simulink model "PVGRIDup2018"  (R2018a)
settings: Solver=VariableStepAuto  StartTime=0.0  StopTime=1  FixedStep=6.17283950617284E-7  MaxStep=2.0E-5  RelTol=1e-3
libraries: powerlib x33, powerlib_meascontrol x5, fuzblock x2, powerlib_extras x2, simulink x2, eePowerMeasurement x1, re_lib x1
(part 1 of 2)
settings Model: Creator=Lenovo  LastModifiedBy=Lenovo
settings SolverCC: AlgebraicLoopSolver=LineSearch
settings DataIOCC: ReturnWorkspaceOutputs=on
settings SFSimCC: SimUseLocalCustomCode=on
settings RTWCC: RTWUseLocalCustomCode=on

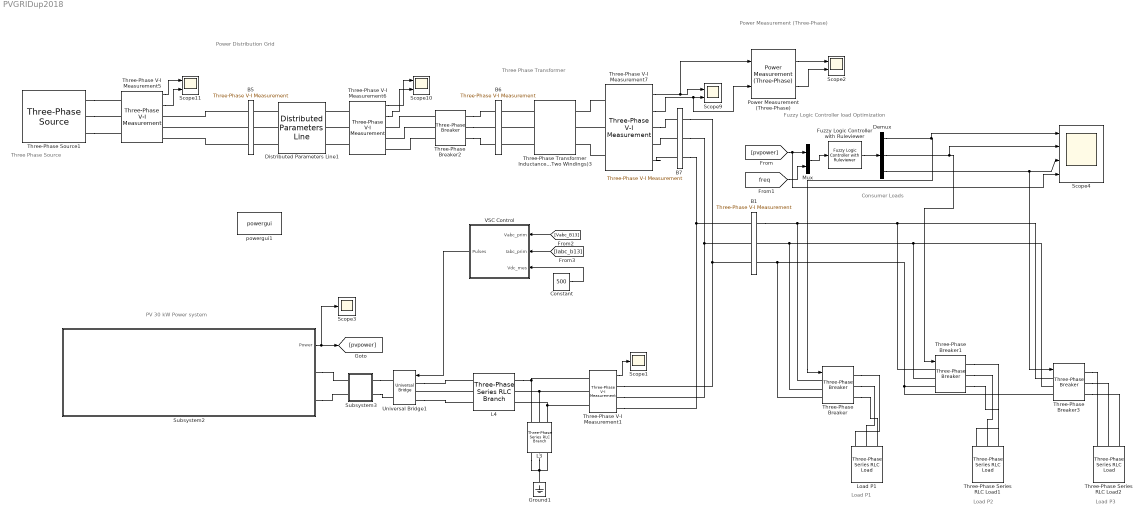
== system PVGRIDup2018 ==
  note: Fuzzy Logic Controller load Optimization
  note: Power Measurement
      | (Three-Phase)
  note: Three Phase Transformer
  note: Three Phase Source
  note: PV 30 kW Power system
  note: Load P1
  note: Power Distribution Grid
  note: Load P2
  note: Load P3
  note: Consumer Loads
  B1 : powerlib/Measurements/Three-Phase V-I Measurement  VoltageMeasurement=no  SetLabelV=off  LabelV=Vabc_B13  Vpu=off  VpuLL=off  CurrentMeasurement=no  SetLabelI=off  LabelI=Iabc_b13  Ipu=off  Pbase=100e6  Vbase=440  OutputType=Magnitude  PhasorSimulation=off  PSBequivalent=0
  B5 : powerlib/Measurements/Three-Phase V-I Measurement  VoltageMeasurement=no  SetLabelV=off  LabelV=Vabc_B12  Vpu=off  VpuLL=off  CurrentMeasurement=no  SetLabelI=off  LabelI=A1  Ipu=off  Pbase=100e6  Vbase=25e3  OutputType=Magnitude  PhasorSimulation=off  PSBequivalent=0
  B6 : powerlib/Measurements/Three-Phase V-I Measurement  VoltageMeasurement=no  SetLabelV=off  LabelV=Vabc_B12  Vpu=off  VpuLL=off  CurrentMeasurement=no  SetLabelI=off  LabelI=A1  Ipu=off  Pbase=100e6  Vbase=440  OutputType=Magnitude  PhasorSimulation=off  PSBequivalent=0
  B7 : powerlib/Measurements/Three-Phase V-I Measurement  VoltageMeasurement=phase-to-ground  SetLabelV=on  LabelV=Vabc_B13  Vpu=off  VpuLL=off  CurrentMeasurement=yes  SetLabelI=on  LabelI=Iabc_b13  Ipu=off  Pbase=100e6  Vbase=440  OutputType=Magnitude  PhasorSimulation=off  PSBequivalent=0
  Constant : Constant  Value=500
  Demux : Demux  Outputs=3
  Distributed Parameters Line1 : powerlib/Elements/Distributed Parameters Line  Phases=3  Frequency=50  Resistance=[0.01273 0.3864]  Inductance="[0.9337e-3  4.1264e-3]"  Capacitance=[12.74e-9 7.751e-9]  Length=100  x1=[-0.000566 5.83136712290493e-10 21736.6395103712 -60787.0989053576;-0.000565 5.82440364018513e-10 21755.7352677324 -60780.2671390469;-0.000564 5.81743958261973e-10 21774.8288778885 -60773.4293739643;-0.000563 5.81047495089606e-10 21793.9203389552 -60766.5856107847;-0.000562 5.8035097457015e-10 21813.0096490482 -60759.7358501836;-0.000561 5.7965439677235e-10 21832.0968062834 -60752.8800928369;-0.00056 5.78957761764954e-10 21851.1818087771 -60746.0183394214;-0.000559 5.78261069616718e-10 21870.2646546456 -60739.1505906142;-0.000558 5.77564320396403e-10 21889.3453420055 -60732.2768470932;-0.000557 5.76867514172774e-10 21908.4238689736 -60725.3971095368;-0.000556 5.76170651014605e-10 21927.500233667 -60718.511378624;-0.000555 5.75473730990671e-10 21946.5744342028 -60711.6196550343;-0.000554 5.74776754169758e-10 21965.6464686987 -60704.721939448;-0.000553 5.74079720620653e-10 21984.7163352721 -60697.8182325458;-0.000552 5.73382630412152e-10 22003.784032041 -60690.9085350092;-0.000551 5.72685483613053e-10 22022.8495571235 -60683.99284752;-0.00055 5.71988280292163e-10 22041.9129086378 -60677.0711707608;-0.000549 5.71291020518294e-10 22060.9740847026 -60670.1435054148;-0.000548 5.70593704360261e-10 22080.0330834366 -60663.2098521657;-0.000547 5.69896331886887e-10 22099.0899029586 -60656.2702116979;-0.000546 5.69198903167e-10 22118.1445413879 -60649.3245846961;-0.000545 5.68501418269433e-10 22137.1969968438 -60642.372971846;-0.000544 5.67803877263027e-10 22156.2472674461 -60635.4153738336;-0.000543 5.67106280216624e-10 22175.2953513143 -60628.4517913457;-0.000542 5.66408627199075e-10 22194.3412465687 -60621.4822250694;-0.000541 5.65710918279236e-10 22213.3849513294 -60614.5066756928;-0.00054 5.65013153525967e-10 22232.4264637169 -60607.5251439041;-0.000539 5.64315333008136e-10 22251.4657818518 -60600.5376303926;-0.000538 5.63617456794614e-10 22270.5029038552 -60593.5441358477;-0.000537 5.6291952495428e-10 22289.537827848 -60586.5446609599;-0.000536 5.62221537556016e-10 22308.5705519516 -60579.5392064197;-0.000535 5.61523494668711e-10 22327.6010742876 -60572.5277729188;-0.000534 5.60825396361258e-10 22346.6293929778 -60565.510361149;-0.000533 5.60127242702558e-10 22365.655506144 -60558.4869718031;-0.000532 5.59429033761516e-10 22384.6794119085 -60551.457605574;-0.000531 5.58730769607041e-10 22403.7011083937 -60544.4222631557;-0.00053 5.5803245030805e-10 22422.7205937223 -60537.3809452425;-0.000529 5.57334075933465e-10 22441.7378660171 -60530.3336525293;-0.000528 5.56635646552211e-10 22460.7529234011 -60523.2803857117;-0.000527 5.55937162233222e-10 22479.7657639977 -60516.2211454858;-0.000526 5.55238623045434e-10 22498.7763859304 -60509.1559325483;-0.000525 5.54540029057792e-10 22517.7847873228 -60502.0847475966;-0.000524 5.53841380339242e-10 22536.7909662991 -60495.0075913285;-0.000523 5.5314267695874e-10 22555.7949209832 -60487.9244644425;-0.000522 5.52443918985244e-10 22574.7966494996 -60480.8353676377;-0.000521 5.5174510648772e-10 22593.7961499729 -60473.7403016137;-0.00052 5.51046239535136e-10 22612.7934205279 -60466.6392670709;-0.000519 5.50347318196469e-10 22631.7884592897 -60459.53226471;-0.000518 5.496483425407e-10 22650.7812643835 -60452.4192952325;-0.000517 5.48949312636813e-10 22669.7718339348 -60445.3003593405;-0.000516 5.48250228553802e-10 22688.7601660693 -60438.1754577364;-0.000515 5.47551090360663e-10 22707.746258913 -60431.0445911236;-0.000514 5.46851898126397e-10 22726.730110592 -60423.9077602058;-0.000513 5.46152651920013e-10 22745.7117192326 -60416.7649656874;-0.000512 5.45453351810523e-10 22764.6910829615 -60409.6162082733;-0.000511 5.44753997866946e-10 22783.6681999055 -60402.4614886692;-0.00051 5.44054590158304e-10 22802.6430681915 -60395.3008075811;-0.000509 5.43355128753627e-10 22821.615685947 -60388.1341657157;-0.000508 5.42655613721949e-10 22840.5860512992 -60380.9615637805;-0.000507 5.41956045132309e-10 22859.554162376 -60373.7830024833;-0.000506 5.41256423053752e-10 22878.5200173052 -60366.5984825326 ...(+32961 chars)]  x2=[-0.000566 3.58367798971719e-09 21848.8110670649 -61151.5428268991;-0.000565 3.58079247310706e-09 21868.0213123234 -61144.6758028705;-0.000564 3.57790660308688e-09 21887.2293992947 -61137.8027441044;-0.000563 3.57502037994147e-09 21906.435326083 -61130.9236512791;-0.000562 3.5721338039557e-09 21925.6390907929 -61124.0385250735;-0.000561 3.56924687541445e-09 21944.8406915289 -61117.1473661671;-0.00056 3.56635959460267e-09 21964.040126396 -61110.2501752401;-0.000559 3.5634719618053e-09 21983.2373934992 -61103.3469529733;-0.000558 3.56058397730735e-09 22002.4324909439 -61096.4377000478;-0.000557 3.55769564139384e-09 22021.6254168355 -61089.5224171457;-0.000556 3.55480695434986e-09 22040.8161692799 -61082.6011049495;-0.000555 3.5519179164605e-09 22060.0047463829 -61075.6737641422;-0.000554 3.54902852801089e-09 22079.1911462508 -61068.7403954076;-0.000553 3.5461387892862e-09 22098.3753669898 -61061.80099943;-0.000552 3.54324870057165e-09 22117.5574067066 -61054.8555768941;-0.000551 3.54035826215248e-09 22136.737263508 -61047.9041284857;-0.00055 3.53746747431395e-09 22155.9149355011 -61040.9466548906;-0.000549 3.53457633734138e-09 22175.090420793 -61033.9831567957;-0.000548 3.53168485152011e-09 22194.2637174912 -61027.0136348881;-0.000547 3.52879301713552e-09 22213.4348237034 -61020.0380898557;-0.000546 3.52590083447302e-09 22232.6037375375 -61013.0565223871;-0.000545 3.52300830381806e-09 22251.7704571016 -61006.0689331711;-0.000544 3.52011542545612e-09 22270.934980504 -60999.0753228975;-0.000543 3.51722219967272e-09 22290.0973058532 -60992.0756922566;-0.000542 3.5143286267534e-09 22309.257431258 -60985.0700419391;-0.000541 3.51143470698375e-09 22328.4153548274 -60978.0583726366;-0.00054 3.5085404406494e-09 22347.5710746705 -60971.0406850409;-0.000539 3.50564582803598e-09 22366.7245888968 -60964.0169798448;-0.000538 3.50275086942919e-09 22385.8758956158 -60956.9872577414;-0.000537 3.49985556511475e-09 22405.0249929375 -60949.9515194246;-0.000536 3.49695991537841e-09 22424.1718789719 -60942.9097655887;-0.000535 3.49406392050597e-09 22443.3165518293 -60935.8619969288;-0.000534 3.49116758078324e-09 22462.4590096201 -60928.8082141404;-0.000533 3.48827089649608e-09 22481.599250455 -60921.7484179197;-0.000532 3.4853738679304e-09 22500.7372724451 -60914.6826089635;-0.000531 3.4824764953721e-09 22519.8730737015 -60907.6107879691;-0.00053 3.47957877910715e-09 22539.0066523355 -60900.5329556346;-0.000529 3.47668071942154e-09 22558.1380064587 -60893.4491126584;-0.000528 3.4737823166013e-09 22577.2671341829 -60886.3592597398;-0.000527 3.4708835709325e-09 22596.3940336202 -60879.2633975784;-0.000526 3.46798448270121e-09 22615.5187028829 -60872.1615268746;-0.000525 3.46508505219359e-09 22634.6411400833 -60865.0536483293;-0.000524 3.46218527969577e-09 22653.7613433342 -60857.9397626441;-0.000523 3.45928516549397e-09 22672.8793107485 -60850.819870521;-0.000522 3.45638470987441e-09 22691.9950404393 -60843.6939726627;-0.000521 3.45348391312336e-09 22711.10853052 -60836.5620697726;-0.00052 3.45058277552711e-09 22730.2197791042 -60829.4241625546;-0.000519 3.44768129737199e-09 22749.3287843055 -60822.280251713;-0.000518 3.44477947894437e-09 22768.4355442382 -60815.1303379531;-0.000517 3.44187732053065e-09 22787.5400570164 -60807.9744219805;-0.000516 3.43897482241725e-09 22806.6423207545 -60800.8125045013;-0.000515 3.43607198489065e-09 22825.7423335672 -60793.6445862226;-0.000514 3.43316880823734e-09 22844.8400935696 -60786.4706678517;-0.000513 3.43026529274385e-09 22863.9355988766 -60779.2907500966;-0.000512 3.42736143869675e-09 22883.0288476036 -60772.1048336661;-0.000511 3.42445724638263e-09 22902.1198378662 -60764.9129192692;-0.00051 3.42155271608814e-09 22921.2085677802 -60757.7150076159;-0.000509 3.41864784809993e-09 22940.2950354616 -60750.5110994165;-0.000508 3.4157426427047e-09 22959.3792390266 -60743.3011953821;-0.000507 3.4128371001892e-09 22978.4611765918 -60736.0852962241;-0.000506 3.40993122084017e-09 22997.5408462738 -60728.8634026549 ...(+32986 chars)]  x3=[-0.000566 5.56062289169838e-11 55.6303279385759 -232.444239909909;-0.000565 5.56073424095848e-11 55.7033497037751 -232.426751656576;-0.000564 5.56084504139612e-11 55.7763659712741 -232.409240463642;-0.000563 5.56095529300035e-11 55.8493767338664 -232.391706332836;-0.000562 5.5610649957603e-11 55.9223819843462 -232.374149265888;-0.000561 5.56117414966513e-11 55.9953817155082 -232.356569264532;-0.00056 5.56128275470409e-11 56.0683759201476 -232.338966330501;-0.000559 5.56139081086644e-11 56.1413645910601 -232.321340465533;-0.000558 5.56149831814152e-11 56.2143477210421 -232.303691671369;-0.000557 5.56160527651872e-11 56.2873253028904 -232.286019949749;-0.000556 5.56171168598749e-11 56.3602973294024 -232.268325302418;-0.000555 5.56181754653732e-11 56.4332637933761 -232.250607731122;-0.000554 5.56192285815777e-11 56.5062246876099 -232.232867237611;-0.000553 5.56202762083844e-11 56.5791800049029 -232.215103823634;-0.000552 5.56213183456899e-11 56.6521297380548 -232.197317490946;-0.000551 5.56223549933914e-11 56.7250738798656 -232.179508241301;-0.00055 5.56233861513865e-11 56.798012423136 -232.161676076457;-0.000549 5.56244118195735e-11 56.8709453606674 -232.143820998174;-0.000548 5.56254319978511e-11 56.9438726852615 -232.125943008215;-0.000547 5.56264466861187e-11 57.0167943897206 -232.108042108344;-0.000546 5.56274558842762e-11 57.0897104668478 -232.090118300327;-0.000545 5.56284595922238e-11 57.1626209094464 -232.072171585934;-0.000544 5.56294578098625e-11 57.2355257103206 -232.054201966936;-0.000543 5.5630450537094e-11 57.3084248622748 -232.036209445106;-0.000542 5.563143777382e-11 57.3813183581142 -232.018194022221;-0.000541 5.56324195199433e-11 57.4542061906446 -232.000155700058;-0.00054 5.56333957753669e-11 57.5270883526721 -231.982094480397;-0.000539 5.56343665399944e-11 57.5999648370037 -231.964010365022;-0.000538 5.56353318137301e-11 57.6728356364466 -231.945903355717;-0.000537 5.56362915964787e-11 57.7457007438089 -231.927773454269;-0.000536 5.56372458881455e-11 57.818560151899 -231.909620662467;-0.000535 5.56381946886362e-11 57.8914138535259 -231.891444982103;-0.000534 5.56391379978573e-11 57.9642618414994 -231.873246414972;-0.000533 5.56400758157156e-11 58.0371041086296 -231.855024962868;-0.000532 5.56410081421186e-11 58.1099406477273 -231.836780627591;-0.000531 5.56419349769742e-11 58.1827714516037 -231.818513410941;-0.00053 5.56428563201911e-11 58.2555965130708 -231.80022331472;-0.000529 5.56437721716781e-11 58.3284158249411 -231.781910340735;-0.000528 5.56446825313451e-11 58.4012293800275 -231.763574490793;-0.000527 5.5645587399102e-11 58.4740371711436 -231.745215766703;-0.000526 5.56464867748596e-11 58.5468391911037 -231.726834170277;-0.000525 5.56473806585292e-11 58.6196354327224 -231.708429703329;-0.000524 5.56482690500225e-11 58.692425888815 -231.690002367676;-0.000523 5.56491519492518e-11 58.7652105521974 -231.671552165137;-0.000522 5.565002935613e-11 58.837989415686 -231.653079097532;-0.000521 5.56509012705705e-11 58.9107624720979 -231.634583166685;-0.00052 5.56517676924873e-11 58.9835297142507 -231.616064374421;-0.000519 5.56526286217948e-11 59.0562911349624 -231.597522722568;-0.000518 5.5653484058408e-11 59.1290467270519 -231.578958212956;-0.000517 5.56543340022426e-11 59.2017964833384 -231.560370847417;-0.000516 5.56551784532147e-11 59.2745403966419 -231.541760627785;-0.000515 5.56560174112408e-11 59.3472784597828 -231.523127555898;-0.000514 5.56568508762382e-11 59.4200106655821 -231.504471633595;-0.000513 5.56576788481247e-11 59.4927370068615 -231.485792862716;-0.000512 5.56585013268185e-11 59.5654574764431 -231.467091245105;-0.000511 5.56593183122385e-11 59.6381720671498 -231.448366782608;-0.00051 5.56601298043039e-11 59.7108807718048 -231.429619477073;-0.000509 5.56609358029348e-11 59.7835835832323 -231.410849330351;-0.000508 5.56617363080516e-11 59.8562804942565 -231.392056344293;-0.000507 5.56625313195752e-11 59.9289714977027 -231.373240520755;-0.000506 5.56633208374273e-11 60.0016565863965 ...(+32997 chars)]  x4=[-0.000566 -4.87376415829962e-11 80.4323722212456 -225.104025756955;-0.000565 -4.87433637657878e-11 80.5030867662651 -225.078746073964;-0.000564 -4.87490811378023e-11 80.5737933659485 -225.053444176592;-0.000563 -4.87547936984754e-11 80.6444920133172 -225.028120067335;-0.000562 -4.87605014472433e-11 80.7151827013937 -225.002773748693;-0.000561 -4.87662043835426e-11 80.7858654232011 -224.977405223168;-0.00056 -4.87719025068105e-11 80.8565401717631 -224.952014493262;-0.000559 -4.87775958164845e-11 80.9272069401046 -224.926601561484;-0.000558 -4.87832843120029e-11 80.997865721251 -224.901166430339;-0.000557 -4.87889679928042e-11 81.0685165082285 -224.87570910234;-0.000556 -4.87946468583273e-11 81.1391592940642 -224.850229579997;-0.000555 -4.88003209080119e-11 81.209794071786 -224.824727865827;-0.000554 -4.88059901412979e-11 81.2804208344224 -224.799203962345;-0.000553 -4.88116545576258e-11 81.3510395750029 -224.773657872072;-0.000552 -4.88173141564365e-11 81.4216502865576 -224.748089597528;-0.000551 -4.88229689371715e-11 81.4922529621177 -224.722499141237;-0.00055 -4.88286188992726e-11 81.5628475947148 -224.696886505724;-0.000549 -4.88342640421823e-11 81.6334341773816 -224.671251693518;-0.000548 -4.88399043653433e-11 81.7040127031514 -224.645594707148;-0.000547 -4.8845539868199e-11 81.7745831650585 -224.619915549147;-0.000546 -4.88511705501932e-11 81.8451455561378 -224.594214222049;-0.000545 -4.88567964107701e-11 81.9156998694251 -224.568490728391;-0.000544 -4.88624174493746e-11 81.9862460979569 -224.542745070711;-0.000543 -4.88680336654517e-11 82.0567842347706 -224.516977251551;-0.000542 -4.88736450584474e-11 82.1273142729044 -224.491187273453;-0.000541 -4.88792516278076e-11 82.1978362053973 -224.465375138964;-0.00054 -4.88848533729792e-11 82.2683500252889 -224.43954085063;-0.000539 -4.88904502934091e-11 82.33885572562 -224.413684411002;-0.000538 -4.8896042388545e-11 82.4093532994317 -224.387805822631;-0.000537 -4.8901629657835e-11 82.4798427397664 -224.361905088071;-0.000536 -4.89072121007277e-11 82.5503240396669 -224.335982209879;-0.000535 -4.8912789716672e-11 82.6207971921772 -224.310037190613;-0.000534 -4.89183625051175e-11 82.6912621903416 -224.284070032835;-0.000533 -4.89239304655142e-11 82.7617190272056 -224.258080739105;-0.000532 -4.89294935973126e-11 82.8321676958155 -224.232069311991;-0.000531 -4.89350518999636e-11 82.9026081892182 -224.206035754059;-0.00053 -4.89406053729185e-11 82.9730405004614 -224.179980067878;-0.000529 -4.89461540156294e-11 83.0434646225939 -224.15390225602;-0.000528 -4.89516978275485e-11 83.113880548665 -224.127802321059;-0.000527 -4.89572368081287e-11 83.1842882717249 -224.10168026557;-0.000526 -4.89627709568234e-11 83.2546877848248 -224.075536092133;-0.000525 -4.89683002730863e-11 83.3250790810163 -224.049369803326;-0.000524 -4.89738247563717e-11 83.3954621533523 -224.023181401734;-0.000523 -4.89793444061344e-11 83.4658369948861 -223.99697088994;-0.000522 -4.89848592218297e-11 83.5362035986721 -223.970738270531;-0.000521 -4.89903692029131e-11 83.6065619577653 -223.944483546096;-0.00052 -4.8995874348841e-11 83.6769120652217 -223.918206719227;-0.000519 -4.90013746590699e-11 83.7472539140979 -223.891907792517;-0.000518 -4.9006870133057e-11 83.8175874974516 -223.865586768562;-0.000517 -4.90123607702599e-11 83.887912808341 -223.839243649959;-0.000516 -4.90178465701368e-11 83.9582298398254 -223.812878439308;-0.000515 -4.90233275321462e-11 84.0285385849647 -223.786491139212;-0.000514 -4.90288036557471e-11 84.0988390368196 -223.760081752275;-0.000513 -4.90342749403991e-11 84.169131188452 -223.733650281102;-0.000512 -4.90397413855622e-11 84.2394150329241 -223.707196728304;-0.000511 -4.90452029906968e-11 84.3096905632993 -223.680721096491;-0.00051 -4.9050659755264e-11 84.3799577726416 -223.654223388276;-0.000509 -4.90561116787252e-11 84.450216654016 -223.627703606273;-0.000508 -4.90615587605422e-11 84.5204672004882 -223.601161753102;-0.000507 -4.90670010001775e-11 84.5907094051246 -223.57459783138 ...(+33554 chars)]  x5=0.000565541566995743  V1=[0 0 0 1.442e-09 6.456e+04 6.456e+04;0 0 0 314.2 314.2 314.2;1.571 1.571 1.571 -0.8406 0.4129 -1.158]  V2=[0 0 0 6.152e-09 6.494e+04 6.494e+04;0 0 0 314.2 314.2 314.2;1.571 1.571 1.571 -0.9733 0.4126 -1.158]  I1=[0 0 0 3.485e-11 239 239;0 0 0 314.2 314.2 314.2;1.571 1.571 1.571 -2.244 0.3044 -1.266]  I2=[0 0 0 3.246e-11 239 239;0 0 0 314.2 314.2 314.2;1.571 1.571 1.571 0.613 0.4126 -1.158]  nHarmo=2  Measurements=None
      settings: SourceProductName=Simscape Power Systems
  Fuzzy Logic Controller with Ruleviewer : fuzblock/Fuzzy Logic  Controller  with Ruleviewer  fismatrix=Pload  Ts=0.1
  Ground1 : powerlib/Elements/Ground  LConnTagsString=a
      settings: SourceProductName=Simscape Electrical
  L3 : powerlib/Elements/Three-Phase Series RLC Branch  LConnTagsString=A|B|C  RConnTagsString=A|B|C  BranchType=C  Resistance=500e-6*377/50/2  Inductance=1e-2  Capacitance=100e-6  Measurements=None
  L4 : powerlib/Elements/Three-Phase Series RLC Branch  LConnTagsString=A|B|C  RConnTagsString=A|B|C  BranchType=RL  Resistance=1  Inductance=3e-2  Capacitance=900e-6  Measurements=None
  Load P1 : powerlib/Elements/Three-Phase Series RLC Load  LConnTagsString=A|B|C  Configuration=Y (grounded)  NominalVoltage=400  Vabc=[1e3 1e3 1e3]  Vabcp=[1e3 1e3 1e3]  NominalFrequency=50  UnbalancedPower=off  ActivePower=10e3  InductivePower=100  CapacitivePower=0  Pabc=[10e3 9e3 11e3]  QLabc=[100 90 110]  QCabc=[100 90 110]  Pabcp=[10e3 9e3 11e3]  QLabcp=[100 90 110]  QCabcp=[100 90 110]  Measurements=None  LoadType=constant Z
      settings: SourceProductName=Simscape Electrical
  Mux : Mux  Inputs=2
  Power Measurement (Three-Phase) : eePowerMeasurement/Power Measurement (Three-Phase)  OverrideUsingVariant=Continuous  F=60  K=[0 1 2 3]  Seq=Positive  Ts=0
      settings: SourceProductName=Simscape Electrical  SourceProductBaseCode=PS
  Scope1 : Scope
  Scope{2,9..11} (4 alike) : Scope  NumInputPorts=2
  Scope3 : Scope
  Scope4 : Scope  NumInputPorts=4
  Subsystem2 : Subsystem
  Subsystem3 : Subsystem
  Three-Phase Series RLC Load1 : powerlib/Elements/Three-Phase Series RLC Load  LConnTagsString=A|B|C  Configuration=Y (grounded)  NominalVoltage=400  Vabc=[1e3 1e3 1e3]  Vabcp=[1e3 1e3 1e3]  NominalFrequency=50  UnbalancedPower=off  ActivePower=10e3  InductivePower=100  CapacitivePower=0  Pabc=[10e3 9e3 11e3]  QLabc=[100 90 110]  QCabc=[100 90 110]  Pabcp=[10e3 9e3 11e3]  QLabcp=[100 90 110]  QCabcp=[100 90 110]  Measurements=None  LoadType=constant Z
      settings: SourceProductName=Simscape Electrical
  Three-Phase Series RLC Load2 : powerlib/Elements/Three-Phase Series RLC Load  LConnTagsString=A|B|C  Configuration=Y (grounded)  NominalVoltage=400  Vabc=[1e3 1e3 1e3]  Vabcp=[1e3 1e3 1e3]  NominalFrequency=50  UnbalancedPower=off  ActivePower=10e3  InductivePower=100  CapacitivePower=0  Pabc=[10e3 9e3 11e3]  QLabc=[100 90 110]  QCabc=[100 90 110]  Pabcp=[10e3 9e3 11e3]  QLabcp=[100 90 110]  QCabcp=[100 90 110]  Measurements=None  LoadType=constant Z
      settings: SourceProductName=Simscape Electrical
  Three-Phase V-I Measurement1 : powerlib/Measurements/Three-Phase V-I Measurement  VoltageMeasurement=phase-to-phase  SetLabelV=off  LabelV=Vabc  Vpu=off  VpuLL=off  CurrentMeasurement=no  SetLabelI=off  LabelI=Iabc  Ipu=off  Pbase=100e6  Vbase=500e3  OutputType=Complex  PhasorSimulation=off  PSBequivalent=0
      settings: SourceProductName=Simscape Electrical
  Three-Phase V-I Measurement5 : powerlib/Measurements/Three-Phase V-I Measurement  VoltageMeasurement=phase-to-ground  SetLabelV=off  LabelV=Vabc  Vpu=off  VpuLL=off  CurrentMeasurement=yes  SetLabelI=off  LabelI=Iabc  Ipu=off  Pbase=100e6  Vbase=500e3  OutputType=Complex  PhasorSimulation=off  PSBequivalent=0
  Three-Phase V-I Measurement6 : powerlib/Measurements/Three-Phase V-I Measurement  VoltageMeasurement=phase-to-ground  SetLabelV=off  LabelV=Vabc  Vpu=off  VpuLL=off  CurrentMeasurement=yes  SetLabelI=off  LabelI=Iabc  Ipu=off  Pbase=100e6  Vbase=500e3  OutputType=Complex  PhasorSimulation=off  PSBequivalent=0
  Three-Phase V-I Measurement7 : powerlib/Measurements/Three-Phase V-I Measurement  VoltageMeasurement=phase-to-phase  SetLabelV=off  LabelV=Vabc_b1  Vpu=off  VpuLL=off  CurrentMeasurement=yes  SetLabelI=off  LabelI=Iabc_b1  Ipu=off  Pbase=100e6  Vbase=500e3  OutputType=Complex  PhasorSimulation=off  PSBequivalent=0
  Three-Phase Breaker : powerlib/Elements/Three-Phase Breaker  InitialState=open  SwitchA=on  SwitchB=on  SwitchC=on  SwitchTimes="[1/60  5/60]"  External=on  BreakerResistance=0.01  SnubberResistance=1e6  SnubberCapacitance=inf  Measurements=None
      settings: SourceProductName=Simscape Electrical
  Three-Phase Breaker1 : powerlib/Elements/Three-Phase Breaker  InitialState=open  SwitchA=on  SwitchB=on  SwitchC=on  SwitchTimes="[1/60  5/60]"  External=on  BreakerResistance=0.01  SnubberResistance=1e6  SnubberCapacitance=inf  Measurements=None
      settings: SourceProductName=Simscape Electrical
  Three-Phase Breaker2 : powerlib/Elements/Three-Phase Breaker  InitialState=closed  SwitchA=off  SwitchB=off  SwitchC=off  SwitchTimes="[1/50  20/50]"  External=off  BreakerResistance=0.001  SnubberResistance=1e6  SnubberCapacitance=inf  Measurements=None
  Three-Phase Breaker3 : powerlib/Elements/Three-Phase Breaker  InitialState=open  SwitchA=on  SwitchB=on  SwitchC=on  SwitchTimes="[1/60  5/60]"  External=on  BreakerResistance=0.01  SnubberResistance=1e6  SnubberCapacitance=inf  Measurements=None
      settings: SourceProductName=Simscape Electrical
  Three-Phase Source1 : powerlib/Electrical Sources/Three-Phase Source  InternalConnection=Yg  VoltagePhases=off  Voltage=63510.4  PhaseAngle=0  Voltage_phases=[25e3 25e3 25e3]/sqrt(3)  PhaseAngles_phases=[0 -120 +120]  Frequency=50  NonIdealSource=on  SpecifyImpedance=on  Resistance=0.8929  Inductance=16.58e-3  ShortCircuitLevel=100e6  BaseVoltage=63510.4  XRratio=7  BusType=swing  Pref=0  Qref=0  Prefabc=[10e3, 10e3, 10e3]  Qrefabc=[0, 0, 0]  Qmin=-inf  Qmax=inf
  Three-Phase Transformer Inductance Matrix Type (Two Windings)3 : powerlib/Elements/Three-Phase Transformer Inductance Matrix Type (Two Windings)  CoreType=Three-limb or five-limb core  Winding1Connection=Yg  Winding2Connection=Yg  AutoTransformer=off  Measurements=None  NominalPower=[100e3 50]  VLLnom=[63510.4 254.03]  WindingResistances=[0.01 0.01]  NoLoadIexcPos=2  NoLoadPlossPos=1000  ShortCircuitReactancePos=0.06  ShortCircuitReactancePosAuto=0.06  NoLoadIexcZero=100  NoLoadPlossZero=1500  ShortCircuitReactanceZero=0.03  ShortCircuitReactanceZeroAuto=0.03
      settings: SourceProductName=Simscape Power Systems  SourceProductBaseCode=PS
  Universal Bridge1 : powerlib/Power Electronics/Universal Bridge  Arms=3  SnubberResistance=1e5  SnubberCapacitance=inf  Device=MOSFET / Diodes  Ron=1e-3  Lon=0  ForwardVoltages="[  0  0  ]"  ForwardVoltage=0  GTOparameters=[ 10e-6 , 20e-6 ]  IGBTparameters=[ 1e-6 , 2e-6 ]  Measurements=None  Measurements_2=None  converterType=Rectifier
      settings: SourceProductName=Simscape Electrical
  VSC Control : Subsystem  mask(VSC Main Controller){nom=[ 100e3  50 ], Vnom=[ 440 440 ], Vnom_dc=440, RLxfo=[0.002  0.06 ], RLchoke=[2e-3  250e-6  ], K_VDCreg=[7  800], K_Ireg=[0.3 20], Ts=50e-6}
      mask prompts: nom "Nominal power and frequency [ Pnom(VA)  Fnom(Hz) ]:"; Vnom "Nominal primary and secondary voltages (Vrms LL) [ Vnom_prim   Vnom_sec ]:"; Vnom_dc "Nominal DC bus voltage (V):"; RLxfo "Total transformer leakage impedance (pu/Pnom) [ Rxfo  Lxf ]"; RLchoke "Choke impedance [ R(ohm) L(H) ]"; K_VDCreg "VDC regultator gains [ Kp  Ki ]:"; K_Ireg "Current regulator gains [ Kp  Ki ]:"; Ts "Sample time"
      mask init:
      | Pnom=nom(1);
      | Fnom=nom(2);
      | Vnom_prim=Vnom(1);
      | Vnom_sec=Vnom(2);
      | Zbase=Vnom_sec^2/Pnom;
      | Rtot_pu=RLxfo(1) + RLchoke(1)/Zbase;
      | Ltot_pu=RLxfo(2) + RLchoke(2)/(Zbase/(2*pi*Fnom));
      | Kp_VDCreg=K_VDCreg(1);
      | Ki_VDCreg=K_VDCreg(2);
      | Kp_Ireg=K_Ireg(1);
      | Ki_Ireg=K_Ireg(2);
      | Vdc_ref=Vnom_dc;
      | % Used to determine initial value of Boost Control (MPPT)
      | assignin('base','Vdc_ref_Inv',Vdc_ref);
  powergui1 : powerlib/powergui  Priority=1  SimulationMode=Discrete  SampleTime=1e-6  frequency=60  Iterations=50  frequencyindice=50  Pbase=100e6  ErrMax=1e-4  UnitsV=kV  UnitsW=MW  buscounter=0  FunctionMessages=off  echomessages=off  EnableUseOfTLC=off  CurrentSourceSwitches=off  DisableSnubberDevices=off  DisableRonSwitches=off  DisableVfSwitches=off  DisplayEquations=off  AutomaticDiscreteSolvers=off  SolverType=Tustin/Backward Euler (TBE)  Interpol=off  ExternalGateDelay=off  methode=off  Ts=100  x0status=blocks  SPID=on  SwTol=0  HookPort=off  NonlinearTolerance=0  nMaxIteration=15  ContinueOnMaxIteration=off  RestoreLinks=warning  ResistiveCurrentMeasurement=off  Frange=[0:2:500]  Ylog=off  Xlog=on  ShowGrid=off  save=off  variable=ZData  structure=0  ZoomFFT=off  StartTime=0.0  cycles=1  DisplayStyle=1  fundamental=60  FreqAxis=off  MaxFrequency=1000  frequencyindicesteady=1  RmsSteady=1  display=off
      settings: SourceProductName=Simscape Electrical
  wires:
  Three-Phase V-I Measurement5/2 -> Scope11/2
  Three-Phase V-I Measurement5/1 -> Scope11/1
  Three-Phase V-I Measurement7/1 -> Power Measurement (Three-Phase)/1, Scope9/1
  Three-Phase V-I Measurement6/2 -> Scope10/2
  Three-Phase V-I Measurement6/1 -> Scope10/1
  [Vabc_B13] -> VSC Control/1(Vabc_prim)
  [Iabc_b13] -> VSC Control/2(Iabc_prim)
  Constant/1 -> VSC Control/3(Vdc_mes)
  VSC Control/1(Pulses) -> Universal Bridge1/1
  Three-Phase V-I Measurement1/1 -> Scope1/1
  Three-Phase V-I Measurement7/2 -> Power Measurement (Three-Phase)/2, Scope9/2
  Power Measurement (Three-Phase)/1 -> Scope2/1
  Power Measurement (Three-Phase)/2 -> Scope2/2
  Mux/1 -> Fuzzy Logic Controller with Ruleviewer/1
  Fuzzy Logic Controller with Ruleviewer/1 -> Demux/1
  Demux/1 -> Scope4/1, Three-Phase Breaker/1
  Demux/2 -> Scope4/2, Three-Phase Breaker1/1
  Subsystem2/1(Power) -> Scope3/1, [pvpower]
  [pvpower] -> Scope4/4, Mux/1
  [freq] -> Mux/2
  Demux/3 -> Three-Phase Breaker3/1, Scope4/3
  connections:
  B5/RConn2 -- Three-Phase V-I Measurement5/RConn2
  Three-Phase Breaker2/LConn2 -- B6/RConn2
  Three-Phase Source1/RConn2 -- Three-Phase V-I Measurement5/LConn2
  Three-Phase V-I Measurement7/RConn3 -- B7/RConn3
  B5/RConn1 -- Three-Phase V-I Measurement5/RConn1
  Three-Phase V-I Measurement6/LConn1 -- Distributed Parameters Line1/RConn1
  Three-Phase Breaker2/RConn3 -- Three-Phase V-I Measurement6/RConn3
  Three-Phase V-I Measurement7/LConn3 -- Three-Phase Transformer Inductance Matrix Type (Two Windings)3/RConn3
  Three-Phase V-I Measurement7/LConn2 -- Three-Phase Transformer Inductance Matrix Type (Two Windings)3/RConn2
  Three-Phase Transformer Inductance Matrix Type (Two Windings)3/LConn2 -- B6/LConn2
  Three-Phase Breaker2/LConn1 -- B6/RConn1
  Three-Phase Source1/RConn3 -- Three-Phase V-I Measurement5/LConn3
  Three-Phase V-I Measurement7/RConn2 -- B7/RConn2
  B5/RConn3 -- Three-Phase V-I Measurement5/RConn3
  Three-Phase V-I Measurement6/LConn3 -- Distributed Parameters Line1/RConn3
  Distributed Parameters Line1/LConn2 -- B5/LConn2
  Three-Phase Breaker2/RConn2 -- Three-Phase V-I Measurement6/RConn2
  Distributed Parameters Line1/LConn3 -- B5/LConn3
  Three-Phase V-I Measurement6/LConn2 -- Distributed Parameters Line1/RConn2
  Distributed Parameters Line1/LConn1 -- B5/LConn1
  Three-Phase Source1/RConn1 -- Three-Phase V-I Measurement5/LConn1
  Three-Phase V-I Measurement7/RConn1 -- B7/RConn1
  Three-Phase Breaker2/RConn1 -- Three-Phase V-I Measurement6/RConn1
  Three-Phase Transformer Inductance Matrix Type (Two Windings)3/LConn1 -- B6/LConn1
  Three-Phase Breaker2/LConn3 -- B6/RConn3
  Three-Phase Transformer Inductance Matrix Type (Two Windings)3/LConn3 -- B6/LConn3
  Three-Phase V-I Measurement7/LConn1 -- Three-Phase Transformer Inductance Matrix Type (Two Windings)3/RConn1
  B7/LConn3 -- Three-Phase V-I Measurement1/RConn3 -- B1/RConn1
  B7/LConn2 -- Three-Phase V-I Measurement1/RConn2 -- B1/RConn2
  B7/LConn1 -- Three-Phase V-I Measurement1/RConn1 -- B1/RConn3
  L3/LConn3 -- Three-Phase V-I Measurement1/LConn3 -- L4/RConn3
  L3/LConn1 -- L4/RConn1 -- Three-Phase V-I Measurement1/LConn1
  L3/LConn2 -- Three-Phase V-I Measurement1/LConn2 -- L4/RConn2
  L3/RConn1 -- Ground1/LConn1 -- L3/RConn3 -- L3/RConn2
  L4/LConn2 -- Universal Bridge1/LConn2
  Universal Bridge1/LConn3 -- L4/LConn3
  Subsystem3/RConn1 -- Universal Bridge1/RConn1
  Subsystem3/RConn2 -- Universal Bridge1/RConn2
  Universal Bridge1/LConn1 -- L4/LConn1
  Subsystem2/RConn1 -- Subsystem3/LConn1
  Subsystem2/RConn2 -- Subsystem3/LConn2
  Three-Phase Breaker/RConn1 -- Load P1/LConn1
  Three-Phase Breaker/RConn2 -- Load P1/LConn2
  Three-Phase Breaker/RConn3 -- Load P1/LConn3
  Three-Phase Breaker1/RConn3 -- Three-Phase Series RLC Load1/LConn3
  Three-Phase Breaker1/RConn1 -- Three-Phase Series RLC Load1/LConn1
  Three-Phase Breaker1/RConn2 -- Three-Phase Series RLC Load1/LConn2
  Three-Phase Breaker3/RConn1 -- Three-Phase Series RLC Load2/LConn1
  Three-Phase Breaker3/RConn3 -- Three-Phase Series RLC Load2/LConn3
  Three-Phase Breaker3/RConn2 -- Three-Phase Series RLC Load2/LConn2
  B1/LConn1 -- Three-Phase Breaker/LConn1 -- Three-Phase Breaker1/LConn1 -- Three-Phase Breaker3/LConn1
  Three-Phase Breaker3/LConn2 -- Three-Phase Breaker1/LConn2 -- Three-Phase Breaker/LConn2 -- B1/LConn2
  Three-Phase Breaker3/LConn3 -- Three-Phase Breaker/LConn3 -- B1/LConn3 -- Three-Phase Breaker1/LConn3
